simulink model "CAVE_MachE"  (R2024a)
settings: configuration reference "ConfigSetDesktopFixedStep" (kept outside this file)
PreLoadFcn:
  | VSS_BICYCLE=Simulink.Variant('Dual=0');
  | VSS_DUAL=Simulink.Variant('Dual=1');
  | Dual=1;
  | load('DriveCycle2.mat')
PostLoadFcn:
  | if any(exist('dsrtsu_mdlpostloadfcn', 'file') ~= 0), dsrtsu_mdlpostloadfcn('Execute', bdroot); end
InitFcn:
  | , if any(exist('rtifpga_mdlclblib', 'file') ~= 0), rtifpga_mdlclblib('Init', bdroot); end,
  | , if any(exist('dsmpb_private', 'file') ~= 0), dsmpb_private('dsmpb_mdlclblib', 'Init', bdroot); end,
  | load('DriveCycle2.mat')
model workspace (MAT data in the model file):
  Gas = 0.383333333333
undefined symbols (not defined in the file or in its folder): AccelCmd, ActTqLF_Nm_, ActTqLR_Nm_, ActTqRF_Nm_, ActTqRR_Nm_, BattChargeLimitMaxPwr, BattChargeLimitSocBpts, BattChargeLimitTbl, BattChrgCapcty, BattDischargeLimitSocBpts, BattDischargeLimitTbl, BattDischargeMaxPwr, BattNumCellsParallel, BattNumCellsSeries, BattOpenVoltCapBpts, BattOpenVoltTbl, BattResistSocBpts, BattResistTbl, BattResistTempBpts, BrakeMaxPrs, BrakeMaxTrq, ChassisDistCg2FrontAxle, ChassisDistCg2RearAxle, ChassisVehMass, CltchCmd, CoastDown, DecelCmd, DiffRatio, DiscIntNeverNeededParam, EnvGravCnst, EnvPrs, EnvTemp, FuelSpecificGrav, GearCmd, h, InitStates, lgSw, limitedMCT, MCT, MtrEffSpdBpts, MtrEffTbl, MtrEffTrqBpts, MtrPwrMax, MtrTrqMax, pMCT, Ref_speed, Ref_time, SteeringCmd, SupvsryCtrlRegenBrkCutOffTbl, SupvsryCtrlRegenSpdBpts, TestScnrioCycleNum, US06, VEH
libraries: VSIGenLib x65, simulink x54, etargetslib x38, dsmpblib x24, vehdynlibtire x12, autolibshared x9, vehdynlibsuspension x7, vehdynlibtirecommon x7, autolibutils x5, CarMaker4SL x4, VsrLibWheel x4, autolibpowerinfoutils x3
(part 3 of 14)

== system CAVE_MachE/Vehicle Under Test/Vehicle/Actuation and Outputs/Vehicle Accel Pedal Voltage Output ==
  APP_pct : Inport
  APP1Tbl : Lookup_n-D  NumberOfTableDimensions=1  BreakpointsForDimension1=[0 100]  Table=[16 78.8]  InternalRulePriority=Speed  RndMeth=Simplest
  APP2Tbl : Lookup_n-D  NumberOfTableDimensions=1  BreakpointsForDimension1=[0 100]  Table=[8 39.4]  InternalRulePriority=Speed  RndMeth=Simplest
  AccelPosition Bypass Enable : Constant  Value=0
  AccelPosition Manual Bypass [%] : Constant  Value=0
  Gain : Gain
  Gain1 : Gain
  Gain2 : Gain
  Gain3 : Gain  Gain=1/100
  Gain4 : Gain  Gain=1/100
  Product2 : Product
  Product3 : Product
  Rate Limiter : RateLimiter  RisingSlewLimit=50  FallingSlewLimit=-50  SampleTimeMode=inherited
  Switch2 : Switch  Criteria=u2 > Threshold  SaturateOnIntegerOverflow=off  InputSameDT=off
  Terminator2 : Terminator
  VRef : Constant  Value=5.01
  Voltage Out (1) : dsmpblib/Data Outport  Priority=-10000
      settings: SourceProductName=dSPACE Model Interface Package for Simulink (MIPS)
  Voltage Out (2) : dsmpblib/Data Outport  Priority=-10000
      settings: SourceProductName=dSPACE Model Interface Package for Simulink (MIPS)
  wires:
  Switch2/1 -> APP1Tbl/1, APP2Tbl/1, Gain2/1  "APP_CmdFinal_pct"
  APP_pct/1 -> Switch2/3
  AccelPosition Manual Bypass [%]/1 -> Rate Limiter/1
  AccelPosition Bypass Enable/1 -> Switch2/2
  Gain/1 -> Voltage Out (2)/1  "APP2_CmdFinal_V"
  Gain1/1 -> Voltage Out (1)/1  "APP1_CmdFinal_V"
  Gain2/1 -> Terminator2/1  "AccelPedal_CmdFinal_pct"
  Rate Limiter/1 -> Switch2/1
  VRef/1 -> Product2/2, Product3/1
  Gain4/1 -> Product3/2
  Product2/1 -> Gain1/1
  APP2Tbl/1 -> Gain4/1
  Gain3/1 -> Product2/1
  Product3/1 -> Gain/1
  APP1Tbl/1 -> Gain3/1

== system CAVE_MachE/Vehicle Under Test/Vehicle/Battery/Battery ==
  note: Thermal model is needed to estimated battery temperature. Ambient temperture is assumed.
  Bus Creator1 : BusCreator  Inputs=1
  Bus Selector : BusSelector  OutputSignals=BattSoc
  Bus Selector2 : BusSelector  OutputSignals=Curr
  Constant : Constant  Value=EnvTemp
  Lithium Ion Battery Pack1 : Subsystem  AncestorBlock=autolibdatasheetbattery/Datasheet Battery  mask(Datasheet Battery){CapacityCtrl=Parameter, OutputVlt=Unfiltered, BattChargeMax=BattChrgCapcty, Em=BattOpenVoltTbl, CapLUTBp=BattOpenVoltCapBpts, RInt=BattResistTbl, BattTempBp=BattResistTempBpts, CapSOCBp=BattResistSocBpts, Ns=BattNumCellsSeries, Np=BattNumCellsParallel, BattCapInit=InitStates(TestScnrioCycleNum).BattSoc*BattChrgCapcty, Tc=1/1000, Vinit=3.75*72, RefBlkName='autolibdatasheetbattery/Datasheet Battery'}
      mask prompts: CapacityCtrl "autoblks:autoblkDatasheetBattery:blkPrm_CapacityCtrl"; OutputVlt "autoblks:autoblkDatasheetBattery:blkPrm_OutputVlt"; BattChargeMax "autoblks:autoblkDatasheetBattery:blkPrm_BattChargeMax"; Em "autoblks:autoblkDatasheetBattery:blkPrm_Em"; CapLUTBp "autoblks:autoblkDatasheetBattery:blkPrm_CapLUTBp"; RInt "autoblks:autoblkDatasheetBattery:blkPrm_RInt"; BattTempBp "autoblks:autoblkDatasheetBattery:blkPrm_BattTempBp"; CapSOCBp "autoblks:autoblkDatasheetBattery:blkPrm_CapSOCBp"; Ns "autoblks:autoblkDatasheetBattery:blkPrm_Ns"; Np "autoblks:autoblkDatasheetBattery:blkPrm_Np"; BattCapInit "autoblks:autoblkDatasheetBattery:blkPrm_BattCapInit"; Tc "autoblks:autoblkDatasheetBattery:blkPrm_Tc"; Vinit "autoblks:autoblkDatasheetBattery:blkPrm_Vinit"
      mask help: autoblks:autoblkDatasheetBattery:blkDesc
      mask init:
      | autoicon('autolibdatasheetbattery',gcb,'Initialization');
      mask Help: eval('autoblkshelp(''pbbatterydatasheet'')');
      mask TypeOptions CapacityCtrl: autoblks:autoblkDatasheetBattery:blkCmb_CapacityCtrlExternalInput | autoblks:autoblkDatasheetBattery:blkCmb_CapacityCtrlParameter
      mask TypeOptions OutputVlt: autoblks:autoblkDatasheetBattery:blkCmb_OutputVltFiltered | autoblks:autoblkDatasheetBattery:blkCmb_OutputVltUnfiltered
      mask DialogControl Container3 Prompt: autoblks:autoblkDatasheetBattery:blkDlg_Container3
      mask DialogControl CapacityCtrl Prompt: Initial battery capacity:
      mask DialogControl OutputVlt Prompt: Output battery voltage:
      mask DialogControl ParameterGroupVar Prompt: autoblks:autoblkDatasheetBattery:blkDlg_ParameterGroupVar
      mask DialogControl BattChargeMax Prompt: Rated capacity at nominal temperature, BattChargeMax [Ah]:
      mask DialogControl Em Prompt: Open circuit voltage table data, Em [V]:
      mask DialogControl CapLUTBp Prompt: Open circuit voltage breakpoints 1, CapLUTBp []:
      mask DialogControl RInt Prompt: Internal resistance table data, RInt [Ohms]:
      mask DialogControl BattTempBp Prompt: Battery temperature breakpoints 1, BattTempBp [K]:
      mask DialogControl CapSOCBp Prompt: Battery capacity breakpoints 2, CapSOCBp []:
      mask DialogControl Ns Prompt: Number of cells in series, Ns []:
      mask DialogControl Np Prompt: Number of cells in parallel, Np []:
      mask DialogControl BattCapInit Prompt: Initial battery capacity, BattCapInit [Ah]:
      mask DialogControl Tc Prompt: Output battery voltage time constant, Tc [s]:
      mask DialogControl Vinit Prompt: Output battery voltage initial value, Vinit [V]:
      mask Display:
      | IconInfo = autoicon('autolibdatasheetbattery', gcb, 'DrawCommands');
      | 
      | image(IconInfo.image, IconInfo.position);
      | 
      | for i = 1:numel(IconInfo.lconn)
      |     port_label('lconn', i, IconInfo.lconn{i})
      | end
      | 
      | for j = 1:numel(IconInfo.rconn)
      |     port_label('rconn', j, IconInfo.rconn{j})
      | end
      | 
      | for k = 1:numel(IconInfo.input)
      |     port_label('input', k, IconInfo.input{k})
      | end
      | 
      | for m = 1:numel(IconInfo.output)
      |     port_label('output', m, IconInfo.output{m})
      | end
  Two-Way Connection1 : TwoWayConnection
  Batt : PMIOPort  Side=Right
  BattSoc : Outport
  BattCurr : Outport  Port=2  Unit=A
  BattVolt : Outport  Port=3  Unit=V
  wires:
  Bus Selector2/1 -> Lithium Ion Battery Pack1/1(BattCurr), BattCurr/1  "<Curr>"
  Lithium Ion Battery Pack1/2(BattVolt) -> BattVolt/1, Bus Creator1/1  "Volt"
  Bus Creator1/1 -> Two-Way Connection1/1
  Constant/1 -> Lithium Ion Battery Pack1/2(BattTemp)
  Bus Selector/1 -> BattSoc/1  "<BattSoc>"
  Lithium Ion Battery Pack1/1(Info) -> Bus Selector/1
  Two-Way Connection1/1 -> Bus Selector2/1
  connections:
  Batt/RConn1 -- Two-Way Connection1/RConn1

== system CAVE_MachE/Vehicle Under Test/Vehicle/Battery/Subsystem1 ==
  BattSoc : Inport
  BattCurr : Inport  Port=2
  BattVolt : Inport  Port=3
  Bus Creator : BusCreator  Inputs=3
  Batt : Outport
  wires:
  BattSoc/1 -> Bus Creator/1  "BattSoc"
  BattCurr/1 -> Bus Creator/2  "BattCurr"
  Bus Creator/1 -> Batt/1  "Batt"
  BattVolt/1 -> Bus Creator/3  "BattVolt"

== system CAVE_MachE/Vehicle Under Test/Vehicle/Driver and Drive Cycle/Driver and PI with FF Control ==
  Vehicle_Spd_kph : Inport
  Vehicle_SpdDmd_kph : Inport  Port=2
  Bus Creator : BusCreator  Inputs=6
  Constant : Constant
  Memory1 : Memory
  Memory2 : Memory
  SpdSat : Saturate  UpperLimit=190  LowerLimit=-5
  Speed controller set : Subsystem
  km to miles : Gain  Gain=1/1.609344
  DriverBus : Outport
  wires:
  Vehicle_SpdDmd_kph/1 -> Memory1/1
  Constant/1 -> Bus Creator/1  "Drive"
  SpdSat/1 -> Speed controller set/1(RefSpd [km/hr]), km to miles/1, Bus Creator/5  "RefSpd [km/hr]"
  Bus Creator/1 -> DriverBus/1  "DriverBus"
  Vehicle_Spd_kph/1 -> Memory2/1
  km to miles/1 -> Bus Creator/6  "RefSpd [mph]"
  Memory1/1 -> SpdSat/1
  Memory2/1 -> Speed controller set/2(VehSpd)
  Speed controller set/1(Out1) -> Bus Creator/2
  Speed controller set/2(Out2) -> Bus Creator/3
  Speed controller set/3(Out3) -> Bus Creator/4

== system CAVE_MachE/Vehicle Under Test/Vehicle/Driver and Drive Cycle/Get Cycle Clock Time ==
  Cycle Trigger : Inport
  Add1 : Sum  Inputs=+-
  Clock1 : Clock
  Clock2 : Clock
  Data Type Conversion : DataTypeConversion  OutDataTypeStr=double  SaturateOnIntegerOverflow=off  RndMeth=Floor
  Memory4 : Memory
  Switch : Switch  Criteria=u2 > Threshold  SaturateOnIntegerOverflow=off  InputSameDT=off
  tCycle : Outport
  wires:
  Switch/1 -> Add1/2, Memory4/1
  Clock1/1 -> Add1/1
  Clock2/1 -> Switch/3
  Add1/1 -> tCycle/1  "tCycle"
  Memory4/1 -> Switch/1
  Cycle Trigger/1 -> Data Type Conversion/1
  Data Type Conversion/1 -> Switch/2

== system CAVE_MachE/Vehicle Under Test/Vehicle/Front Wheel Drive/Ideal Diff ==
  DrvShfTrq : Inport
  Omega : Inport  Port=2
  Add : Sum
  Add1 : Sum
  Bus Creator1 : BusCreator  Inputs=2
  Bus Creator2 : BusCreator  Inputs=2
  Bus Creator3 : BusCreator  Inputs=2
  Bus Creator4 : BusCreator  Inputs=4
  Bus to Vector : BusToVector
  Constant : Constant  Value=0
  Demux : Demux  Outputs=[2,2]
  Demux1 : Demux  Outputs=2
  Gain1 : Gain  Gain=0.5
  Gain2 : Gain  Gain=DiffRatio
  Gain3 : Gain  Gain=DiffRatio
  Gain4 : Gain  Gain=0.5
  Memory : Memory
  Memory1 : Memory
  Power Bus : Subsystem
  Terminator : Terminator
  Terminator1 : Terminator
  Vector Concatenate : Concatenate  NumInputs=4
  Diff : Outport  VectorParamsAs1DForOutWhenUnconnected=off
  AxlTrq : Outport  Port=2  VectorParamsAs1DForOutWhenUnconnected=off
  PropShaftSpd : Outport  Port=3  VectorParamsAs1DForOutWhenUnconnected=off
  wires:
  Demux1/2 -> [Axl2Spd], Add1/2
  Vector Concatenate/1 -> AxlTrq/1
  Gain4/1 -> [Axl1Trq], Add/1, Vector Concatenate/1, [Axl2Trq], Add/2, Vector Concatenate/2  "T_FL"
  DrvShfTrq/1 -> [DriveshftTrq], Bus to Vector/1
  [DriveshftTrq] -> Power Bus/1(DriveshftTrq), Bus Creator1/1  "DriveshftTrq"
  [Axl1Spd] -> Bus Creator2/2  "Axl1Spd"
  Demux/1 -> Demux1/1
  Add1/1 -> Gain1/1
  Bus Creator4/1 -> Diff/1
  Add/1 -> Terminator/1  "AxlTrqLump"
  [Axl2Trq] -> Bus Creator3/1  "Axl2Trq"
  Omega/1 -> Demux/1
  Memory/1 -> Gain3/1
  Bus to Vector/1 -> Memory/1
  Bus Creator3/1 -> Bus Creator4/3  "Axl2"
  Bus Creator2/1 -> Bus Creator4/2  "Axl1"
  Bus Creator1/1 -> Bus Creator4/1  "Driveshft"
  [DriveshftSpd] -> Bus Creator1/2, Power Bus/2(Speed)  "Speed"
  Gain2/1 -> Memory1/1  "Spd"
  Constant/1 -> Vector Concatenate/4, Vector Concatenate/3  "T_RR"
  Demux1/1 -> [Axl1Spd], Add1/1
  Memory1/1 -> PropShaftSpd/1, [DriveshftSpd]
  Gain3/1 -> Gain4/1
  [Axl1Trq] -> Bus Creator2/1  "Axl1Trq"
  Power Bus/1(PwrInfo) -> Bus Creator4/4
  Gain1/1 -> Gain2/1
  [Axl2Spd] -> Bus Creator3/2  "Axl2Spd"
  Demux/2 -> Terminator1/1

== system CAVE_MachE/Vehicle Under Test/Vehicle/Front Wheel Drive/Ideal Diff AWD ==
  DrvShfTrq : Inport
  Omega : Inport  Port=2
  Add : Sum
  Add1 : Sum  Inputs=++++
  Bus Creator1 : BusCreator  Inputs=2
  Bus Creator2 : BusCreator  Inputs=2
  Bus Creator3 : BusCreator  Inputs=2
  Bus Creator4 : BusCreator  Inputs=4
  Bus to Vector : BusToVector
  Demux : Demux  Outputs=[2,2]
  Demux1 : Demux  Outputs=2
  Demux2 : Demux  Outputs=2
  Gain1 : Gain  Gain=0.25
  Gain2 : Gain  Gain=DiffRatio
  Gain3 : Gain  Gain=DiffRatio
  Gain4 : Gain  Gain=0.25
  Memory : Memory
  Memory1 : Memory
  Power Bus : Subsystem
  Terminator : Terminator
  Vector Concatenate : Concatenate  NumInputs=4
  Diff : Outport  VectorParamsAs1DForOutWhenUnconnected=off
  AxlTrq : Outport  Port=2  VectorParamsAs1DForOutWhenUnconnected=off
  PropShaftSpd : Outport  Port=3  VectorParamsAs1DForOutWhenUnconnected=off
  wires:
  Power Bus/1(PwrInfo) -> Bus Creator4/4
  Demux1/2 -> [Axl2Spd], Add1/2
  Gain4/1 -> [Axl4Trq], Vector Concatenate/4, [Axl3Trq], Vector Concatenate/3, [Axl1Trq], Add/1, Vector Concatenate/1, [Axl2Trq], Add/2, Vector Concatenate/2  "T_RR"
  Demux/2 -> Demux2/1
  Vector Concatenate/1 -> AxlTrq/1
  Gain1/1 -> Gain2/1
  Gain3/1 -> Gain4/1
  [Axl1Trq] -> Bus Creator2/1  "Axl1Trq"
  Bus to Vector/1 -> Memory/1
  Gain2/1 -> Memory1/1  "Spd"
  Memory/1 -> Gain3/1
  Bus Creator2/1 -> Bus Creator4/2  "Axl1"
  Memory1/1 -> PropShaftSpd/1, [DriveshftSpd]
  Demux1/1 -> [Axl1Spd], Add1/1
  [DriveshftSpd] -> Bus Creator1/2, Power Bus/2(Speed)  "Speed"
  Bus Creator4/1 -> Diff/1
  [Axl2Spd] -> Bus Creator3/2  "Axl2Spd"
  Bus Creator1/1 -> Bus Creator4/1  "Driveshft"
  Add/1 -> Terminator/1  "AxlTrqLump"
  [Axl1Spd] -> Bus Creator2/2  "Axl1Spd"
  [Axl2Trq] -> Bus Creator3/1  "Axl2Trq"
  DrvShfTrq/1 -> [DriveshftTrq], Bus to Vector/1
  Demux/1 -> Demux1/1
  Bus Creator3/1 -> Bus Creator4/3  "Axl2"
  [DriveshftTrq] -> Power Bus/1(DriveshftTrq), Bus Creator1/1  "DriveshftTrq"
  Add1/1 -> Gain1/1
  Omega/1 -> Demux/1
  Demux2/1 -> Add1/3
  Demux2/2 -> Add1/4

== system CAVE_MachE/Vehicle Under Test/Vehicle/Front Wheel Drive/Real Diff ==
  DrvShfTrq : Inport
  Omega : Inport  Port=2
  Bus Creator1 : BusCreator  Inputs=2
  Bus Creator2 : BusCreator  Inputs=2
  Bus Creator3 : BusCreator  Inputs=2
  Bus Creator4 : BusCreator  Inputs=4
  Constant : Constant  Value=0
  Demux : Demux  Outputs=[2,2]
  Demux1 : Demux  Outputs=2
  DiffPress : Constant  Value=0
  Limited Slip Differential : autolibshareddiff/Limited Slip Differential  DiffEffModelPopup=Constant  InterpMethod=Linear point-slope  extTamb=off  shaftSwitchMask=To the left of center-line  Ndiff=7.05  Jd=0.025  bd=1e-3  Jw1=0.01  bw1=1e-3  Jw2=0.01  bw2=1e-3  omegaw1o=0  omegaw2o=0  eta=0.98  eta_tbl=reshape([0.64 0.76 0.8 0.81 0.83 0.84 0.84 0.56 0.73 0.78 0.8 0.83 0.84 0.84 0.54 0.71 0.77 0.8 0.82 0.84 0.84 0.53 0.71 0.77 0.8 0.83 0.84 0.84 0.51 0.71 0.77 0.8 0.83 0.84 0.85 0.52 0.7 0.77 0.8 0.83 0.84 0.85 0.51 0.71 0.76 0.79 0.83 0.84 0.85 0.5 0.69 0.76 0.79 0.82 0.84 0.85 0.45 0.68 0.75 0.78 0.82 0.84 0.85 0.43 0.67 0.74 0.78 0.81 0.83 0.84 0.38 0.63 0.71 0.75 0.8 0.82 0.83 0.81 0.86 0.88 0.89 0.89 0.89 0.9 0.77 0.85 0.87 0.88 0.89 0.9 0.9 0.72 0.82 0.86 0.87 0.88 0.89 0.9 0.68 0.8 0.84 0.86 0.88 0.89 0.89 0.67 0.8 0.84 0.86 0.88 0.89 0.9 0.67 0.8 0.84 0.86 0.88 0.89 0.9 0.65 0.8 0.84 0.86 0.88 0.89 0.9 0.64 0.79 0.83 0.86 0.88 0.89 0.9 0.63 0.78 0.83 0.86 0.88 0.89 0.9 0.59 0.76 0.82 0.85 0.87 0.89 0.9 0.53 0.73 0.8 0.83 0.86 0.88 0.89], 7, 11, 2)  Trq_bpts=[25, 50, 75, 100, 150, 200, 250]  omega_bpts=[52.4 78.5 105 131 157 183 209 262 314 419 524]  Temp_bpts=[290 358]  Tamb=297.15  couplingType=Pre-loaded ideal clutch  Ndisks=8  Reff=.08  Fc=1000  muc=[.16 0.13 0.115 0.11 0.105 0.1025 0.10125 .10125]  dw=[0 10 20 40 60 80 100 1000]  Tdw=[-100, -90, -50, -5, 0, 5, 50, 90, 100]  dwT=[-200, -175, -100, - 50, 0, 50, 100, 175, 200]  TTin=[-200 -175 -100 - 50 0 50 100 175 200]  Tin=[-200 -175 -100 - 50 0 50 100 175 200]  tauC=.04  IdealInterpMethod=Linear point-slope  IdealExtrapMethod=Linear  TdwInterpMethod=Flat  TdwExtrapMethod=Clip  TTinInterpMethod=Flat  TTinExtrapMethod=Clip  maxAbsSpd=5e3  aMode=2
      settings: LibrarySourceBlock=vdynlib/Powertrain/Drivetrain/Final Drive Unit/Limited Slip Differential
  Power Bus : Subsystem
  Terminator : Terminator
  Terminator1 : Terminator
  Terminator3 : Terminator
  Torsional Compliance1 : autolibsharedcoupling/Torsional Compliance  port_config=Simulink  extInfo=off  k=10000  b=400  theta_o=0  domega_o=0  omega_c=300  blkID=0  aMode=2
      settings: LibrarySourceBlock=vdynlib/Powertrain/Drivetrain/Couplings/Torsional Compliance
  Torsional Compliance2 : autolibsharedcoupling/Torsional Compliance  port_config=Simulink  extInfo=off  k=10000  b=400  theta_o=0  domega_o=0  omega_c=300  blkID=0  aMode=2
      settings: LibrarySourceBlock=vdynlib/Powertrain/Drivetrain/Couplings/Torsional Compliance
  Vector Concatenate : Concatenate  NumInputs=4
  Vector Concatenate1 : Concatenate  NumInputs=4
  Diff : Outport  VectorParamsAs1DForOutWhenUnconnected=off
  AxlTrq : Outport  Port=2  VectorParamsAs1DForOutWhenUnconnected=off
  PropShaftSpd : Outport  Port=3  VectorParamsAs1DForOutWhenUnconnected=off
  wires:
  Limited Slip Differential/3 -> [Axl1Spd], Torsional Compliance2/1
  Demux1/1 -> Torsional Compliance2/2
  Limited Slip Differential/1 -> Terminator/1
  DrvShfTrq/1 -> [DriveshftTrq], Limited Slip Differential/1
  Limited Slip Differential/4 -> [Axl2Spd], Torsional Compliance1/1
  Demux1/2 -> Torsional Compliance1/2
  Demux/1 -> Demux1/1
  Torsional Compliance1/1 -> Limited Slip Differential/3
  Torsional Compliance2/1 -> Limited Slip Differential/2
  Demux/2 -> Terminator1/1
  Constant/1 -> Vector Concatenate/4, Vector Concatenate/3  "T_RR"
  Torsional Compliance1/2 -> [Axl2Trq], Vector Concatenate/2  "T_FR"
  Torsional Compliance2/2 -> [Axl1Trq], Vector Concatenate/1  "T_FL"
  Omega/1 -> Demux/1
  Vector Concatenate/1 -> AxlTrq/1
  Vector Concatenate1/1 -> Terminator3/1
  DiffPress/1 -> Vector Concatenate1/4, Vector Concatenate1/3, Vector Concatenate1/1, Vector Concatenate1/2
  [DriveshftTrq] -> Power Bus/1(DriveshftTrq), Bus Creator1/1  "DriveshftTrq"
  [Axl1Spd] -> Bus Creator2/2  "Axl1Spd"
  [Axl2Trq] -> Bus Creator3/1  "Axl2Trq"
  Bus Creator4/1 -> Diff/1
  [Axl2Spd] -> Bus Creator3/2  "Axl2Spd"
  [DriveshftSpd] -> Bus Creator1/2, Power Bus/2(Speed)  "Speed"
  Bus Creator1/1 -> Bus Creator4/1  "Driveshft"
  [Axl1Trq] -> Bus Creator2/1  "Axl1Trq"
  Power Bus/1(PwrInfo) -> Bus Creator4/4
  Bus Creator2/1 -> Bus Creator4/2  "Axl1"
  Bus Creator3/1 -> Bus Creator4/3  "Axl2"
  Limited Slip Differential/2 -> [DriveshftSpd], PropShaftSpd/1

== system CAVE_MachE/Vehicle Under Test/Vehicle/Powertrain Supervisory Controller /Engine Torque Command ==
  AccelCmdIn : Inport
  DecelCmdIn : Inport  Port=2
  DriverGearCmdIn : Inport  Port=3
  VehSpd : Inport  Port=4
  BattSoc : Inport  Port=5
  MtrSpd : Inport  Port=6
  Accel Pedal to Traction Wheel Torque Request1 : Subsystem
  Battery Management System : Subsystem
  Motor Torque Arbitration and Power Management : Subsystem
  Series Regen Braking : Subsystem  InitFcn=%[~]=autosharedicon('autolibutils',gcb,0);  VariantControl=Variant
  MtrTrqCmd : Outport
  AccelCmd : Outport  Port=2
  BrkCmd : Outport  Port=3
  DriverGearCmd : Outport  Port=4
  wires:
  DecelCmdIn/1 -> Series Regen Braking/4("DecelCmd ")  "DecelPdl"
  DriverGearCmdIn/1 -> DriverGearCmd/1
  [AccelPdl] -> Motor Torque Arbitration and Power Management/2(AccelPdl)
  MtrSpd/1 -> [MotSpd], Series Regen Braking/3(MotSpd)  "MotSpd"
  AccelCmdIn/1 -> AccelCmd/1, Accel Pedal to Traction Wheel Torque Request1/1(AccelPdl), [AccelPdl]
  VehSpd/1 -> [VehSpd], Series Regen Braking/2(VehSpd)  "VehSpd"
  BattSoc/1 -> Battery Management System/1(SOC), Series Regen Braking/1(BattSoc)  "SOC"
  Battery Management System/1(BattPwrDischrgLmt) -> Motor Torque Arbitration and Power Management/3(BattPwrDisChrgLmt)  "BattPwrDischrgLmt"
  Series Regen Braking/2(" BrkCmd") -> BrkCmd/1  "BrkCmd"
  Battery Management System/2(BattPwrChrgLmt) -> Motor Torque Arbitration and Power Management/4("BattPwrChrgLmt ")  "BattPwrChrgLmt"
  Series Regen Braking/1(" MotTrqCmdRegen") -> Motor Torque Arbitration and Power Management/6(MotTrqCmdRegen)  "MotTrqCmdRegen"
  [MotSpd] -> Motor Torque Arbitration and Power Management/5(MotSpd)
  Motor Torque Arbitration and Power Management/1(MotTrqCmdFinal) -> MtrTrqCmd/1  "MotTrqCmd"
  [VehSpd] -> Accel Pedal to Traction Wheel Torque Request1/2(MotSpd)
  Accel Pedal to Traction Wheel Torque Request1/1(TrqCmd) -> Motor Torque Arbitration and Power Management/1(MotTrqCmdTrac)

== system CAVE_MachE/Vehicle Under Test/Vehicle/Powertrain Supervisory Controller /Subsystem1 ==
  MtrTrqCmd : Inport
  AccelCmd : Inport  Port=2
  BrkCmd : Inport  Port=3
  DriverGearCmd : Inport  Port=4
  SteeringCmd : Inport  Port=5
  Bus Creator : BusCreator  Inputs=5
  SupvsryCtrl : Outport
  wires:
  MtrTrqCmd/1 -> Bus Creator/1  "MtrTrqCmd"
  Bus Creator/1 -> SupvsryCtrl/1  "SupvsryCtrl"
  AccelCmd/1 -> Bus Creator/2  "AccelCmd"
  BrkCmd/1 -> Bus Creator/3  "BrkCmd"
  DriverGearCmd/1 -> Bus Creator/4  "DriverGearCmd"
  SteeringCmd/1 -> Bus Creator/5  "SteeringCmd"

== system CAVE_MachE/Vehicle Under Test/Vehicle/Powertrain Supervisory Controller /Subsystem4 ==
  Driver : Inport
  Chassis : Inport  Port=2
  Batt : Inport  Port=3
  Mtr : Inport  Port=4
  Bus Selector : BusSelector  OutputSignals=AccelCmd,DecelCmd,GearCmd
  Bus Selector1 : BusSelector  OutputSignals=VehSpd
  Bus Selector2 : BusSelector  OutputSignals=BattSoc
  Bus Selector3 : BusSelector  OutputSignals=MtrSpd
  AccelCmd : Outport  VectorParamsAs1DForOutWhenUnconnected=off
  DecelCmd : Outport  Port=2  VectorParamsAs1DForOutWhenUnconnected=off
  DriverGearCmd : Outport  Port=3  VectorParamsAs1DForOutWhenUnconnected=off
  VehSpd : Outport  Port=4  VectorParamsAs1DForOutWhenUnconnected=off
  BattSoc : Outport  Port=5  VectorParamsAs1DForOutWhenUnconnected=off
  MtrSpd : Outport  Port=6  VectorParamsAs1DForOutWhenUnconnected=off
  wires:
  Driver/1 -> Bus Selector/1
  Bus Selector/1 -> AccelCmd/1  "<AccelCmd>"
  Bus Selector/3 -> DriverGearCmd/1  "<GearCmd>"
  Chassis/1 -> Bus Selector1/1
  Bus Selector1/1 -> VehSpd/1  "<VehSpd>"
  Bus Selector/2 -> DecelCmd/1  "<DecelCmd>"
  Batt/1 -> Bus Selector2/1
  Bus Selector2/1 -> BattSoc/1  "<BattSoc>"
  Mtr/1 -> Bus Selector3/1
  Bus Selector3/1 -> MtrSpd/1  "<MtrSpd>"

== system CAVE_MachE/Vehicle Under Test/Vehicle/Rototest and ORNL Interface/DummyPT ==
  WhlSpeedIn : Inport
  APPToTorque : Lookup_n-D  NumberOfTableDimensions=1  BreakpointsForDimension1=[0 100]  Table=[0 184]  InternalRulePriority=Speed  RndMeth=Simplest
  APPToTorque1 : Lookup_n-D  NumberOfTableDimensions=1  BreakpointsForDimension1=[0 100]  Table=[0 184]  InternalRulePriority=Speed  RndMeth=Simplest
  APP_pct : Constant  Value=0
  BPP_pct : Constant  Value=0
  FDR : Gain  Gain=3.18
  Flip : Gain  Gain=-1
  Gear : Product
  Memory : Memory
  NissanTrans : Lookup_n-D  NumberOfTableDimensions=1  BreakpointsForDimension1=[0 5 10 15 25 34 45 55]  Table=[5.25 3.03 1.95 1.46 1.22 1.00 0.81 0.67]  ExtrapMethod=Clip  InternalRulePriority=Speed  RndMeth=Simplest
  Sum : Sum  Inputs=++|
  WheelRadius : Gain  Gain=0.3235
  kph2mph : Gain  Gain=0.621
  mps2kph : Gain  Gain=3.6
  WheelTorqueOut : Outport
  wires:
  kph2mph/1 -> NissanTrans/1  "Speed_mph"
  APPToTorque/1 -> Sum/1  "APPTorque"
  mps2kph/1 -> kph2mph/1  "Speed_kph"
  BPP_pct/1 -> APPToTorque1/1
  NissanTrans/1 -> Gear/2  "Gear"
  Gear/1 -> FDR/1  "TransTorqueOut"
  APPToTorque1/1 -> Flip/1
  Flip/1 -> Sum/2  "BPPTorque"
  APP_pct/1 -> APPToTorque/1
  Sum/1 -> Gear/1  "TorqueTotal"
  WheelRadius/1 -> mps2kph/1  "Speed_mps"
  FDR/1 -> Memory/1  "WheelTorqueOut"
  WhlSpeedIn/1 -> WheelRadius/1
  Memory/1 -> WheelTorqueOut/1

== system CAVE_MachE/Vehicle Under Test/Vehicle/Rototest and ORNL Interface/Format CM Powertrain Signals ==
  note: Can Bypass with my own brake model
  BrakingTorques : Inport
  RotoWheelSpd : Inport  Port=2
  AxlTrq : Inport  Port=3
  MaxRegen : Inport  Port=4
  Bus Creator1 : BusCreator  Inputs=42
  Bus Selector2 : BusSelector  OutputSignals=Brake IF Trq_WB FL,Brake IF Trq_WB FR,Brake IF Trq_WB RL,Brake IF Trq_WB RR
  BusCreator2 : BusCreator  Inputs=42
  Demux : Demux
  Demux1 : Demux  Outputs=42
      settings: DisplayOption=none
  Demux2 : Demux
  Discrete-Time Integrator{4..7} (4 alike) : DiscreteIntegrator  IntegratorMethod=Integration: Backward Euler  SampleTime=0.001  ICPrevOutput=DiscIntNeverNeededParam  ICPrevScaledInput=DiscIntNeverNeededParam
  Gain{5..8} (4 alike) : Gain  Gain=-1
  Ground{2..5} (4 alike) : Ground
  Ignition : Constant
  Memory{1..4} (4 alike) : Memory
  Operation Error : Constant  Value=4
  Operation State Driving : Constant  Value=4
  Product{1..4} (4 alike) : Product  RndMeth=Zero
  Saturation{1..4} (4 alike) : Saturate  UpperLimit=1  LowerLimit=-1
  Zero{1..5} (5 alike) : Constant  Value=0
  PowerTrainOutIdeal : Outport
  wires:
  Saturation4/1 -> Product4/2
  Demux1/3 -> BusCreator2/3  "PT IF OperationError"
  Demux1/2 -> BusCreator2/2  "PT IF OperationState"
  Demux1/40 -> BusCreator2/40  "PT IF WRR Trq_Supp2WC"
  Demux1/9 -> BusCreator2/9  "PT IF Trq_Supp2Bdy1B x"
  Discrete-Time Integrator6/1 -> Bus Creator1/29  "PT WRL rot"
  Demux1/1 -> BusCreator2/1  "PT IF Ignition"
  MaxRegen/1 -> Bus Creator1/28, Bus Creator1/21
  BusCreator2/1 -> PowerTrainOutIdeal/1
  Operation State Driving/1 -> Bus Creator1/2
  Gain8/1 -> Bus Creator1/38
  Demux1/16 -> BusCreator2/16  "PT IF WFL rotv"
  Demux1/21 -> BusCreator2/21  "PT IF WFL Trq_BrakeReg_max"
  Ground2/1 -> Bus Creator1/7
  Demux1/23 -> BusCreator2/23  "PT IF WFR rotv"
  Demux1/14 -> BusCreator2/14  "PT IF DL_iDiff_mean"
  Demux1/4 -> BusCreator2/4  "PT IF GearNo"
  Demux1/17 -> BusCreator2/17  "PT IF WFL Trq_B2W"
  Product3/1 -> Gain5/1
  Demux1/5 -> BusCreator2/5  "PT IF Engine_rotv"
  Demux1/11 -> BusCreator2/11  "PT IF Trq_Supp2Bdy1B z"
  Demux1/12 -> BusCreator2/12  "PT IF Trq_Supp2BdyEng x"
  Demux1/7 -> BusCreator2/7  "PT IF Trq_Supp2Bdy1 y"
  Discrete-Time Integrator5/1 -> Bus Creator1/22  "PT WFR rot"
  Demux1/42 -> BusCreator2/42  "PT IF WRR Trq_BrakeReg_max"
  Gain5/1 -> Bus Creator1/17
  Demux1/18 -> BusCreator2/18  "PT IF WFL Trq_Drive"
  Demux1/8 -> BusCreator2/8  "PT IF Trq_Supp2Bdy1 z"
  Demux1/38 -> BusCreator2/38  "PT IF WRR Trq_B2W"
  Memory4/1 -> Saturation4/1
  Demux1/10 -> BusCreator2/10  "PT IF Trq_Supp2Bdy1B y"
  Demux1/27 -> BusCreator2/27  "PT IF WFR Trq_BrakeReg"
  Demux1/24 -> BusCreator2/24  "PT IF WFR Trq_B2W"
  Demux1/25 -> BusCreator2/25  "PT IF WFR Trq_Drive"
  Demux1/26 -> BusCreator2/26  "PT IF WFR Trq_Supp2WC"
  Demux1/13 -> BusCreator2/13  "PT IF Trq_Supp2BdyEng y"
  Demux1/15 -> BusCreator2/15  "PT IF WFL rot"
  Bus Selector2/2 -> Product1/1  "<Brake IF Trq_WB FR>"
  Memory3/1 -> Saturation3/1
  Demux1/19 -> BusCreator2/19  "PT IF WFL Trq_Supp2WC"
  Demux1/22 -> BusCreator2/22  "PT IF WFR rot"
  Demux1/29 -> BusCreator2/29  "PT IF WRL rot"
  Demux1/33 -> BusCreator2/33  "PT IF WRL Trq_Supp2WC"
  Demux1/30 -> BusCreator2/30  "PT IF WRL rotv"
  Demux1/28 -> BusCreator2/28  "PT IF WFR Trq_BrakeReg_max"
  Demux1/35 -> BusCreator2/35  "PT IF WRL Trq_BrakeReg_max"
  Demux1/39 -> BusCreator2/39  "PT IF WRR Trq_Drive"
  Zero4/1 -> Bus Creator1/33, Bus Creator1/34, Bus Creator1/35
  Demux1/34 -> BusCreator2/34  "PT IF WRL Trq_BrakeReg"
  Demux1/37 -> BusCreator2/37  "PT IF WRR rotv"
  Demux1/31 -> BusCreator2/31  "PT IF WRL Trq_B2W"
  Demux1/32 -> BusCreator2/32  "PT IF WRL Trq_Drive"
  Demux1/36 -> BusCreator2/36  "PT IF WRR rot"
  Zero3/1 -> Bus Creator1/26, Bus Creator1/27
  Demux/4 -> Memory4/1, Discrete-Time Integrator7/1, Bus Creator1/37  "rotv RR"
  Zero2/1 -> Bus Creator1/19, Bus Creator1/20
  Zero1/1 -> Bus Creator1/5, Bus Creator1/4, Bus Creator1/12, Bus Creator1/14, Bus Creator1/13, Bus Creator1/11, Bus Creator1/10, Bus Creator1/9, Bus Creator1/8
  Demux1/20 -> BusCreator2/20  "PT IF WFL Trq_BrakeReg"
  Product2/1 -> Gain7/1
  Discrete-Time Integrator4/1 -> Bus Creator1/15  "PT WFL rot"
  Demux/2 -> Memory1/1, Discrete-Time Integrator5/1, Bus Creator1/23  "rotv FR"
  Discrete-Time Integrator7/1 -> Bus Creator1/36  "PtT WRR rot"
  Zero5/1 -> Bus Creator1/40, Bus Creator1/41, Bus Creator1/42
  Demux1/6 -> BusCreator2/6  "PT IF Trq_Supp2Bdy1 x"
  Demux1/41 -> BusCreator2/41  "PT IF WRR Trq_BrakeReg"
  BrakingTorques/1 -> Bus Selector2/1
  Operation Error/1 -> Bus Creator1/3
  Demux/3 -> Memory2/1, Discrete-Time Integrator6/1, Bus Creator1/30  "rotv RL"
  Memory1/1 -> Saturation1/1
  Ground4/1 -> Bus Creator1/6
  Bus Selector2/1 -> Product3/1  "<Brake IF Trq_WB FL>"
  Gain6/1 -> Bus Creator1/24
  Ignition/1 -> Bus Creator1/1  "PT Ignition"
  Memory2/1 -> Saturation2/1
  Saturation1/1 -> Product1/2
  Bus Selector2/3 -> Product2/1  "<Brake IF Trq_WB RL>"
  Gain7/1 -> Bus Creator1/31
  Demux/1 -> Memory3/1, Discrete-Time Integrator4/1, Bus Creator1/16  "rotv FL"
  Product4/1 -> Gain8/1
  Bus Creator1/1 -> Demux1/1
  Saturation2/1 -> Product2/2
  Product1/1 -> Gain6/1
  Bus Selector2/4 -> Product4/1  "<Brake IF Trq_WB RR>"
  Saturation3/1 -> Product3/2
  RotoWheelSpd/1 -> Demux/1
  AxlTrq/1 -> Demux2/1
  Demux2/1 -> Bus Creator1/18  "TrqDrv FL"
  Demux2/2 -> Bus Creator1/25  "TrqDrv FR"
  Demux2/3 -> Bus Creator1/32  "TrqDrv RL"
  Demux2/4 -> Bus Creator1/39  "TrqDrv RR"

== system CAVE_MachE/Vehicle Under Test/Vehicle/Rototest and ORNL Interface/From Rototest ==
  Input : Inport
  Bus Creator : BusCreator  Inputs=30
  Bus Selector1 : BusSelector  OutputSignals=ActSpLF_rpm,ActSpRF_rpm,ActSpLR_rpm,ActSpRR_rpm
  Mux1 : Mux
  RotoTestEthRX : Subsystem  AncestorBlock=VSIGenLib/RotoTestEthRX
      mask Display:
      | color('white')
      | disp('RotTestEthTx')
      | port_label('output', 1, 'ID')
      | port_label('output', 2, 'ProtocolVer')
      | port_label('output', 3, 'ActTqLF (Nm)')
      | port_label('output', 4, 'RefRR_NmORrpm')
      | port_label('output', 5, 'ActTempLF (C)')
      | port_label('output', 6, 'ActTqRF (Nm)')
      | port_label('output', 7, 'ActSpRF (rpm)')
      | port_label('output', 8, 'ActTempRF (C)')
      | port_label('output', 9, 'ActTqLR (Nm)')
      | port_label('output', 10, 'ActSpLR (rpm)')
      | port_label('output', 11, 'ActTempLR (C)')
      | port_label('output', 12, 'ActTqRR (Nm)')
      | port_label('output', 13, 'ActSpRR (rpm)')
      | port_label('output', 14, 'ActTempRR (Nm)')
      | port_label('output', 15, 'RefLF (Nm)')
      | port_label('output', 16, 'RefRF (rpm)')
      | port_label('output', 17, 'RefLR (Nm)')
      | port_label('output', 18, 'RefRR (Nm)')
      | port_label('output', 19, 'UnitsStatusLF (enum)')
      | port_label('output', 20, 'UnitsStatusRF (enum)')
      | port_label('output', 21, 'UnitsStatusLR (enum)')
      | port_label('output', 22, 'UnitsStatusRR (enum)')
      | port_label('output', 23, 'WatchdogCnt (int)')
      | port_label('output', 24, 'FaultActive (enum)')
      | port_label('output', 25, 'WarningsActive (enum)')
      | port_label('output', 26, 'SpTqRR (enum)')
      | port_label('output', 27, 'SpTqLR (enum)')
      | port_label('output', 28, 'SpTqRF (enum)')
      | port_label('output', 29, 'SpTqLF (enum)')
      | port_label('output', 30, 'SystemActive (bool)')
  SpdAct : Outport
  AxlTrq : Outport  Port=2
  wires:
  RotoTestEthRX/8(ActTempRF_C) -> Bus Creator/8
  RotoTestEthRX/23(WatchdogCnt) -> Bus Creator/23
  RotoTestEthRX/18(RefRR_Nm) -> Bus Creator/18
  Mux1/1 -> SpdAct/1
  RotoTestEthRX/19(UnitsStatusLF) -> Bus Creator/19
  RotoTestEthRX/4(ActSpLF_rpm) -> Bus Creator/4
  Bus Creator/1 -> AxlTrq/1, Bus Selector1/1
  Bus Selector1/4 -> Mux1/4  "<ActSpRR_rpm>"
  RotoTestEthRX/24(FaultActive) -> Bus Creator/24
  RotoTestEthRX/22(UnitsStatusRR) -> Bus Creator/22
  Bus Selector1/3 -> Mux1/3  "<ActSpLR_rpm>"
  RotoTestEthRX/25(WarningsActive) -> Bus Creator/25
  Bus Selector1/1 -> Mux1/1  "<ActSpLF_rpm>"
  Bus Selector1/2 -> Mux1/2  "<ActSpRF_rpm>"
  RotoTestEthRX/5(ActTempLF_C) -> Bus Creator/5
  RotoTestEthRX/30(SystemActive) -> Bus Creator/30
  RotoTestEthRX/20(UnitsStatusRF) -> Bus Creator/20
  RotoTestEthRX/15(RefLF_Nm) -> Bus Creator/15
  RotoTestEthRX/16(RefRF_rpm) -> Bus Creator/16
  RotoTestEthRX/17(RefLR_Nm) -> Bus Creator/17
  RotoTestEthRX/2(ProtocolVer) -> Bus Creator/2
  RotoTestEthRX/7(ActSpRF_rpm) -> Bus Creator/7
  RotoTestEthRX/21(UnitsStatusLR) -> Bus Creator/21
  RotoTestEthRX/11(ActTempLR_C) -> Bus Creator/11
  RotoTestEthRX/1(ID) -> Bus Creator/1
  RotoTestEthRX/28(SpTqRF) -> Bus Creator/28
  RotoTestEthRX/29(SpTqLF) -> Bus Creator/29
  RotoTestEthRX/27(SpTqLR) -> Bus Creator/27
  RotoTestEthRX/26(SpTqRR) -> Bus Creator/26
  RotoTestEthRX/14(ActTempRR_Nm) -> Bus Creator/14
  RotoTestEthRX/3(ActTqLF_Nm) -> Bus Creator/3
  RotoTestEthRX/6(ActTqRF_Nm_) -> Bus Creator/6
  RotoTestEthRX/9(ActTqLR_Nm) -> Bus Creator/9
  RotoTestEthRX/13(ActSpRR_rpm) -> Bus Creator/13
  RotoTestEthRX/10(ActSpLR_rpm) -> Bus Creator/10
  RotoTestEthRX/12(ActTqRR_Nm) -> Bus Creator/12
  Input/1 -> RotoTestEthRX/1(Input)

== system CAVE_MachE/Vehicle Under Test/Vehicle/Rototest and ORNL Interface/Get Wheel Spd Cmd Based on Wheel Dynamics ==
  BrakingTorques : Inport
  Trq_T2W : Inport  Port=2
  AxlTrq : Inport  Port=3
  MaxRegen : Inport  Port=4
  FxIn : Inport  Port=5
  Saturation : Saturate  UpperLimit=100  LowerLimit=0
  Saturation1 : Saturate  UpperLimit=300  LowerLimit=-300
  Scope : Scope
  WheelSpdCmd : Subsystem
  Whl Dynamics & Format CM Powertrain Signal : Subsystem
  WhlSpdCmd : Outport
  wires:
  Whl Dynamics & Format CM Powertrain Signal/1(PowerTrainOutIdeal) -> WheelSpdCmd/1(In1)
  BrakingTorques/1 -> Whl Dynamics & Format CM Powertrain Signal/1(BrakingTorques)
  Trq_T2W/1 -> Whl Dynamics & Format CM Powertrain Signal/2(Trq_T2W)
  MaxRegen/1 -> Whl Dynamics & Format CM Powertrain Signal/4(MaxRegen)
  AxlTrq/1 -> Whl Dynamics & Format CM Powertrain Signal/3(AxlTrq)
  FxIn/1 -> Whl Dynamics & Format CM Powertrain Signal/5(FxIn)
  [SimOmega] -> Scope/1, Saturation/1
  Saturation/1 -> WhlSpdCmd/1

== system CAVE_MachE/Vehicle Under Test/Vehicle/Rototest and ORNL Interface/RotoTrqPreprocess ==
  AxleTrqRaw : Inport
  Bus Selector1 : BusSelector  OutputSignals=ActTqLF_Nm_,ActTqRF_Nm_,ActTqLR_Nm_,ActTqRR_Nm_
  Compare To Constant : simulink/Logic and Bit Operations/Compare To Constant  relop=>=  const=-15  OutDataTypeStr=boolean
  Compare To Constant1 : simulink/Logic and Bit Operations/Compare To Constant  relop=<=  const=0  OutDataTypeStr=boolean
  Data Type Conversion{1..4} (4 alike) : DataTypeConversion  OutDataTypeStr=double  SaturateOnIntegerOverflow=off  RndMeth=Floor
  FirstOrderFilterTau{,1..3} (4 alike) : VSIGenLib/FirstOrderFilterTau  SystemSampleTime=-1  VariantActivationTime=update diagram  AllowFlexibleInterface=on  Latency=0  AutoFrameSizeCalculation=off
  Ground : Ground
  Logical Operator : Logic  AllPortsSameDT=off  OutDataTypeStr=boolean
  ManualTrq_Nm : Constant  Value=0
  Mux : Mux
  Mux1 : Mux
  SatTrq : Saturate  UpperLimit=1000  LowerLimit=-1000
  Tau : Constant  Value=0.01
  TorqueIn : Switch  Criteria=u2 > Threshold  SaturateOnIntegerOverflow=off  InputSameDT=off
  "TorqueIn " : Switch  Criteria=u2 > Threshold  SaturateOnIntegerOverflow=off  InputSameDT=off
  AxleTrqRoto : Outport
  AxleTrqVeh : Outport  Port=2
  wires:
  Mux/1 -> AxleTrqRoto/1, TorqueIn/1
  ManualTrq_Nm/1 -> Mux1/4, Mux1/3, Mux1/2, Mux1/1
  Tau/1 -> FirstOrderFilterTau/2, FirstOrderFilterTau1/2, FirstOrderFilterTau2/2, FirstOrderFilterTau3/2
  Ground/1 -> "TorqueIn "/1
  Logical Operator/1 -> "TorqueIn "/2
  Data Type Conversion4/1 -> Mux/4  "RR"
  Data Type Conversion3/1 -> Mux/3  "LR"
  Mux1/1 -> TorqueIn/3
  [Switch] -> TorqueIn/2
  Bus Selector1/4 -> FirstOrderFilterTau3/1  "<ActTqRR_Nm_>"
  Compare To Constant/1 -> Logical Operator/1
  Bus Selector1/3 -> FirstOrderFilterTau2/1  "<ActTqLR_Nm_>"
  Bus Selector1/2 -> FirstOrderFilterTau1/1  "<ActTqRF_Nm_>"
  TorqueIn/1 -> SatTrq/1
  "TorqueIn "/1 -> AxleTrqVeh/1  "Trq"
  FirstOrderFilterTau1/1 -> Data Type Conversion2/1
  Data Type Conversion2/1 -> Mux/2  "RF"
  AxleTrqRaw/1 -> Bus Selector1/1
  FirstOrderFilterTau/1 -> Data Type Conversion1/1
  FirstOrderFilterTau3/1 -> Data Type Conversion4/1
  Bus Selector1/1 -> FirstOrderFilterTau/1  "<ActTqLF_Nm_>"
  Compare To Constant1/1 -> Logical Operator/2
  SatTrq/1 -> "TorqueIn "/3, Compare To Constant1/1, Compare To Constant/1
  FirstOrderFilterTau2/1 -> Data Type Conversion3/1
  Data Type Conversion1/1 -> Mux/1  "LF"

== system CAVE_MachE/Vehicle Under Test/Vehicle/Rototest and ORNL Interface/Subsystem2 ==
  AxlTorq : Inport
  BusCreator1 : BusCreator  Inputs=16
  BusCreator2 : BusCreator  Inputs=16
  Constant : Constant  Value=0
  Constant1 : Constant  Value=0
  Demux : Demux  Outputs=16
      settings: DisplayOption=none
  Terminator : Terminator
  Zero1 : Constant  Value=0
  Zero2 : Constant  Value=0
  Zero5 : Constant  Value=0
  BrakeUpd : Outport
  wires:
  Demux/9 -> BusCreator1/9  "Brake IF Trq_Reg_trg FL"
  Demux/6 -> BusCreator1/6  "Brake IF Trq_PB FR"
  Constant1/1 -> BusCreator2/1, BusCreator2/2  "Brake IF Trq_WB FL"
  Demux/14 -> BusCreator1/14  "Brake IF Trq_DriveSrc_trg d1"
  Zero2/1 -> BusCreator2/16, BusCreator2/15, BusCreator2/14, BusCreator2/13  "Brake IF Trq_DriveSrc_trg d3"
  Demux/11 -> BusCreator1/11  "Brake IF Trq_Reg_trg RL"
  Demux/15 -> BusCreator1/15  "Brake IF Trq_DriveSrc_trg d2"
  Demux/2 -> BusCreator1/2  "Brake IF Trq_WB FR"
  Demux/16 -> BusCreator1/16  "Brake IF Trq_DriveSrc_trg d3"
  Zero1/1 -> BusCreator2/12, BusCreator2/11, BusCreator2/10, BusCreator2/9  "Brake IF Trq_Reg_trg RR"
  Demux/4 -> BusCreator1/4  "Brake IF Trq_WB RR"
  Demux/3 -> BusCreator1/3  "Brake IF Trq_WB RL"
  Constant/1 -> BusCreator2/4, BusCreator2/3  "Brake IF Trq_WB RL"
  BusCreator1/1 -> BrakeUpd/1
  Demux/1 -> BusCreator1/1  "Brake IF Trq_WB FL"
  Demux/8 -> BusCreator1/8  "Brake IF Trq_PB RR"
  Demux/10 -> BusCreator1/10  "Brake IF Trq_Reg_trg FR"
  BusCreator2/1 -> Demux/1
  Demux/13 -> BusCreator1/13  "Brake IF Trq_DriveSrc_trg d0"
  Demux/5 -> BusCreator1/5  "Brake IF Trq_PB FL"
  Demux/7 -> BusCreator1/7  "Brake IF Trq_PB RL"
  Zero5/1 -> BusCreator2/8, BusCreator2/7, BusCreator2/6, BusCreator2/5  "Brake IF Trq_PB RR"
  Demux/12 -> BusCreator1/12  "Brake IF Trq_Reg_trg RR"
  AxlTorq/1 -> Terminator/1

== system CAVE_MachE/Vehicle Under Test/Vehicle/Rototest and ORNL Interface/To Rototest with Band-Aid ==
  note: Torque Model: Low speed
      | Speed Model: Normal speed
  note: OutMode = 0 is Torque
      | OutMode = 1 is Speed
  note: Switch = 0 Overides
      | Switch = 1 Model
  SpeedCmd_rps : Inport
  AxleTrq_roto_Nm : Inport  Port=2
  BRAKE_PRESSED : Inport  Port=3
  Vehicle_Speed_kph : Inport  Port=4
  Band-Aid : Subsystem
  Demux : Demux
  Demux1 : Demux
  Demux2 : Demux
  Logging : Subsystem  Commented=on
  MasterSw : Constant  Value=0
  Mode Override : Subsystem
  ModeOut : Switch  Criteria=u2 > Threshold  SaturateOnIntegerOverflow=off  InputSameDT=off
  ModeSwitch : MultiPortSwitch  DataPortOrder=Zero-based contiguous  Inputs=2  zeroidx=on  SaturateOnIntegerOverflow=off  InputSameDT=off
  Mux2 : Mux
  Mux4 : Mux
  Mux5 : Mux
  RateLimSpd : RateLimiter  RisingSlewLimit=500  FallingSlewLimit=-500  SampleTimeMode=inherited
  RotoTestEthTx : Subsystem  AncestorBlock=VSIGenLib/RotoTestEthTx
      mask Display:
      | color('white')
      | disp('RotTestEthTx')
      | port_label('input', 1, 'RefLF_NmORrpm')
      | port_label('input', 2, 'RefRF_NmORrpm')
      | port_label('input', 3, 'RefLR_NmORrpm')
      | port_label('input', 4, 'RefRR_NmORrpm')
      | port_label('input', 5, 'SqTrRR')
      | port_label('input', 6, 'SqTrLR')
      | port_label('input', 7, 'SqTrRF')
      | port_label('input', 8, 'SqTrLF')
      | port_label('input', 9, 'SystemActive')
      | port_label('output', 1, 'Status (bool)')
      | port_label('output', 2, 'Sent Bytes (int)')
  SatSpd : Saturate  UpperLimit=500  LowerLimit=0
  Scope : Scope
  SpeedOut : Switch  Criteria=u2 > Threshold  SaturateOnIntegerOverflow=off  InputSameDT=off
  SystemActive : Constant  Value=0  OutDataTypeStr=uint8
  Transfer Fcn{,1..3} (4 alike) : TransferFcn  Denominator=[0.02 1]
  TrqSpd Override : Subsystem
  ZeroTorque : Constant  Value=0  OutDataTypeStr=uint8
  rads2rpm : Gain  Gain=9.5492965964254
  Out1 : Outport
  tag scope: Switch=global
  wires:
  Mux4/1 -> ModeSwitch/2
  Demux/3 -> Mux2/3  "LRIn"
  Demux1/4 -> Transfer Fcn3/1
  Demux/2 -> Mux2/2  "RFIn"
  MasterSw/1 -> [Switch]
  TrqSpd Override/1(Ovr) -> SpeedOut/3
  ZeroTorque/1 -> Mux4/2, Mux4/3, Mux4/4, Mux4/1
  Demux/1 -> Mux2/1  "LFIn"
  SpeedOut/1 -> RateLimSpd/1
  RateLimSpd/1 -> SatSpd/1
  rads2rpm/1 -> Demux/1
  ModeSwitch/1 -> Scope/1, Demux1/1
  Demux/4 -> Mux2/4  "RRIn"
  Band-Aid/1(OutMode) -> Mux5/4, Mux5/3, Mux5/2, Mux5/1, ModeSwitch/1
  ModeOut/1 -> Demux2/1
  [Switch] -> SpeedOut/2
  SatSpd/1 -> ModeSwitch/3  "Spd"
  [Switch] -> ModeOut/2
  Mux5/1 -> ModeOut/1
  Demux2/1 -> RotoTestEthTx/5(SpTqRR)
  Demux1/3 -> Transfer Fcn2/1
  Demux2/3 -> RotoTestEthTx/7(SpTqRF)
  Demux2/2 -> RotoTestEthTx/6(SpTqLR)
  SystemActive/1 -> RotoTestEthTx/9(SystemActive)
  RotoTestEthTx/1(Output) -> Out1/1  "ByteSend"
  Demux1/1 -> Transfer Fcn/1
  Demux1/2 -> Transfer Fcn1/1
  Demux2/4 -> RotoTestEthTx/8(SpTqLF)
  SpeedCmd_rps/1 -> rads2rpm/1
  Mode Override/1(Ovr) -> ModeOut/3
  AxleTrq_roto_Nm/1 -> Band-Aid/2(InTrq_Nm)
  Mux2/1 -> Band-Aid/1(InSpd_rpm)
  Band-Aid/2(OutSpd_rpm) -> SpeedOut/1
  BRAKE_PRESSED/1 -> Band-Aid/3(BRAKE_PRESSED)
  Vehicle_Speed_kph/1 -> Band-Aid/4(VehSpd_kph)
  Transfer Fcn/1 -> RotoTestEthTx/1(RefLF_NmORrpm)
  Transfer Fcn1/1 -> RotoTestEthTx/2(RefRF_NmORrpm)
  Transfer Fcn2/1 -> RotoTestEthTx/3(RefLR_NmORrpm)
  Transfer Fcn3/1 -> RotoTestEthTx/4(RefRR_NmORrpm)

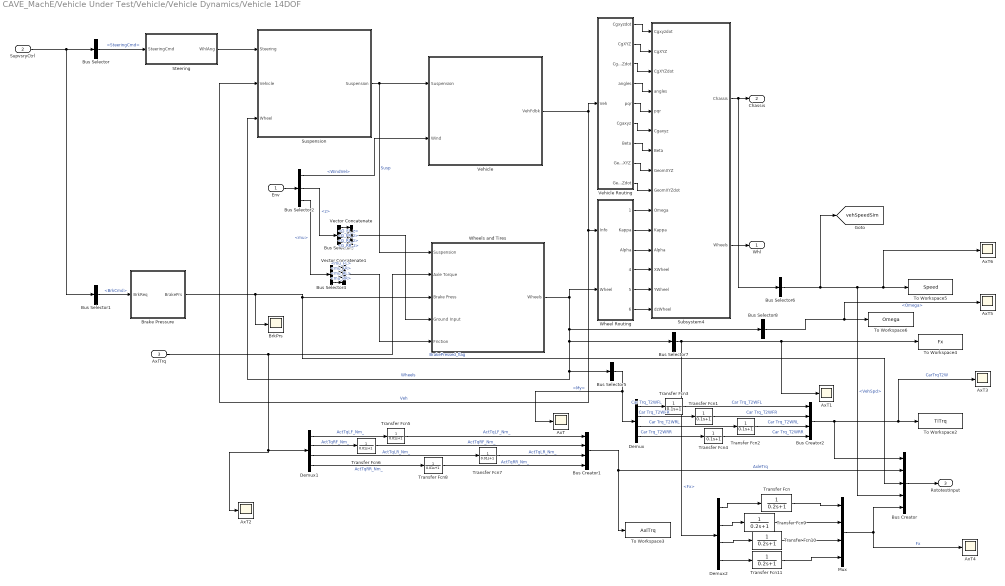
== system CAVE_MachE/Vehicle Under Test/Vehicle/Vehicle Dynamics/Vehicle 14DOF ==
  Env : Inport
  SupvsryCtrl : Inport  Port=2
  AxlTrq : Inport  Port=3
  AxT{,1..6} (7 alike) : Scope
  Brake Pressure : Subsystem
  BrkPrs : Scope
  Bus Creator : BusCreator  Inputs=5
  Bus Creator1 : BusCreator  Inputs=ActTqLF_Nm_,ActTqRF_Nm_,ActTqLR_Nm_,ActTqRR_Nm_
  Bus Creator2 : BusCreator  Inputs=Car Trq_T2WFL,Car Trq_T2WFR,Car Trq_T2WRL,Car Trq_T2WRR
  Bus Selector : BusSelector  OutputSignals=SteeringCmd
  Bus Selector1 : BusSelector  OutputSignals=BrkCmd
  Bus Selector2 : BusSelector  OutputSignals=WindVel,GndBus.z,GndBus.mu
  Bus Selector3 : BusSelector  OutputSignals=G_FL_z,G_FR_z,G_RL_z,G_RR_z
  Bus Selector4 : BusSelector  OutputSignals=mu_FL,mu_FR,mu_RL,mu_RR
  Bus Selector5 : BusSelector  OutputSignals=TireFrame.My
  Bus Selector6 : BusSelector  OutputSignals=VehSpd
  Bus Selector7 : BusSelector  OutputSignals=TireFrame.Fx
  Bus Selector8 : BusSelector  OutputSignals=TireFrame.Omega
  Demux : Demux
  Demux1 : Demux
  Demux2 : Demux
  Mux : Mux
  Steering : Subsystem
  Subsystem4 : Subsystem
  Suspension : Subsystem  Variant=on  VariantControlMode=label  LabelModeActiveChoice=3
      mask Display:
      | switch str2num(get_param(gcb,'ActiveVariant'))
      |     case 1
      |         image('suspdw.png');
      |     case 2
      |         image([imread('suspindmap.png');imread('suspsamap.png')]);
      |     case 3
      |          image([imread('suspmacp.png');imread('suspsacoil.png')]);
      |     case 4
      |          image('suspmacp.png');
      |     case 5
      |          image('suspindmap.png');
      | end
  To Workspace2 : ToWorkspace  VariableName=TiTrq  SampleTime=-1
      settings: Save2DSignal=2-D array (concatenate along first dimension)
  To Workspace3 : ToWorkspace  VariableName=AxlTrq  SampleTime=-1
      settings: Save2DSignal=2-D array (concatenate along first dimension)
  To Workspace4 : ToWorkspace  VariableName=Fx  SampleTime=-1
      settings: Save2DSignal=2-D array (concatenate along first dimension)
  To Workspace5 : ToWorkspace  VariableName=Speed  SampleTime=-1
      settings: Save2DSignal=2-D array (concatenate along first dimension)
  To Workspace6 : ToWorkspace  VariableName=Omega  SampleTime=-1
      settings: Save2DSignal=2-D array (concatenate along first dimension)
  Transfer Fcn{,9..11} (4 alike) : TransferFcn  Denominator=[0.2 1]
  Transfer Fcn{1..4} (4 alike) : TransferFcn  Denominator=[0.1 1]
  Transfer Fcn{5..8} (4 alike) : TransferFcn  Denominator=[0.01 1]
  Vector Concatenate : Concatenate  NumInputs=4
  Vector Concatenate1 : Concatenate  NumInputs=4
  Vehicle : Subsystem
      mask Display: image('6dofcar.png');
  Vehicle Routing : Subsystem
  Wheel Routing : Subsystem
  Wheels and Tires : Subsystem
      mask Display: image('wheel3dof.png')
  Whl : Outport
  Chassis : Outport  Port=2
  RototestInput : Outport  Port=3
  tag scope: vehSpeedSim=global
  wires:
  Vehicle Routing/9(GeomXYZdot) -> Subsystem4/9(GeomXYZdot)
  Vehicle Routing/8(GeomXYZ) -> Subsystem4/8(GeomXYZ)
  Vehicle Routing/1(Cgxyzdot) -> Subsystem4/1(Cgxyzdot)
  Vehicle Routing/5(pqr) -> Subsystem4/5(pqr)
  Vehicle Routing/4(angles) -> Subsystem4/4(angles)
  Vehicle Routing/3(CgXYZdot) -> Subsystem4/3(CgXYZdot)
  Vehicle Routing/7(Beta) -> Subsystem4/7(Beta)
  Wheels and Tires/1(Wheels) -> Wheel Routing/2(Wheel), Bus Selector7/1, Bus Selector5/1, Suspension/3(Wheel), Bus Selector8/1  "Wheels"
  Vehicle Routing/2(CgXYZ) -> Subsystem4/2(CgXYZ)
  Vehicle/1(VehFdbk) -> Suspension/2(Vehicle), Wheel Routing/1(Info), Vehicle Routing/1(Veh)  "Veh"
  Suspension/1(Suspension) -> Vehicle/1(Suspension), Wheels and Tires/1(Suspension)  "Susp"
  Bus Selector2/1 -> Vehicle/2(Wind)  "<WindVel>"
  Steering/1(WhlAng) -> Suspension/1(Steering)
  Bus Selector/1 -> Steering/1(SteeringCmd)  "<SteeringCmd>"
  SupvsryCtrl/1 -> Bus Selector/1, Bus Selector1/1
  Bus Selector1/1 -> Brake Pressure/1(BrkReq)  "<BrkCmd>"
  Env/1 -> Bus Selector2/1
  Vehicle Routing/6(Cgaxyz) -> Subsystem4/6(Cgaxyz)
  Wheel Routing/1(Omega) -> Subsystem4/10(Omega)
  Wheel Routing/3(Alpha) -> Subsystem4/12(Alpha)
  Wheel Routing/4(XWheel) -> Subsystem4/13(XWheel)
  Wheel Routing/2(Kappa) -> Subsystem4/11(Kappa)
  Wheel Routing/5(YWheel) -> Subsystem4/14(YWheel)
  Wheel Routing/6(ZWheel) -> Subsystem4/15(dzWheel)
  Subsystem4/2(Wheels) -> Whl/1
  AxlTrq/1 -> Demux1/1, AxT2/1, Wheels and Tires/2(Axle Torque)
  Bus Selector2/2 -> Bus Selector3/1  "<z>"
  Bus Selector3/1 -> Vector Concatenate/1  "<G_FL_z>"
  Bus Selector3/2 -> Vector Concatenate/2  "<G_FR_z>"
  Bus Selector3/3 -> Vector Concatenate/3  "<G_RL_z>"
  Bus Selector3/4 -> Vector Concatenate/4  "<G_RR_z>"
  Vector Concatenate/1 -> Wheels and Tires/4(Ground Input)
  Bus Selector4/4 -> Vector Concatenate1/4  "<mu_RR>"
  Bus Selector2/3 -> Bus Selector4/1  "<mu>"
  Bus Selector4/3 -> Vector Concatenate1/3  "<mu_RL>"
  Bus Selector4/2 -> Vector Concatenate1/2  "<mu_FR>"
  Bus Selector4/1 -> Vector Concatenate1/1  "<mu_FL>"
  Vector Concatenate1/1 -> Wheels and Tires/5(Friction)
  Bus Selector6/1 -> [vehSpeedSim], Bus Creator/4, AxT6/1, To Workspace5/1  "<VehSpd>"
  Brake Pressure/1(BrakePrs) -> BrkPrs/1, Bus Creator/3, Wheels and Tires/3(Brake Press)  "BrakePressed_flag"
  Bus Creator1/1 -> To Workspace3/1, Bus Creator/2  "AxleTrq"
  Bus Creator2/1 -> Bus Creator/1, AxT3/1, To Workspace2/1  "CarTrqT2W"
  Bus Selector5/1 -> Demux/1, AxT/1  "<My>"
  Subsystem4/1(Chassis) -> Bus Selector6/1, Chassis/1
  Bus Selector7/1 -> Demux2/1, AxT1/1, To Workspace4/1  "<Fx>"
  Bus Selector8/1 -> AxT5/1, To Workspace6/1  "<Omega>"
  Bus Creator/1 -> RototestInput/1
  Transfer Fcn5/1 -> Bus Creator1/1  "ActTqLF_Nm_"
  Demux1/3 -> Transfer Fcn7/1  "ActTqLR_Nm_"
  Transfer Fcn8/1 -> Bus Creator1/4  "ActTqRR_Nm_"
  Demux1/2 -> Transfer Fcn6/1  "ActTqRF_Nm_"
  Transfer Fcn6/1 -> Bus Creator1/2  "ActTqRF_Nm_"
  Demux1/1 -> Transfer Fcn5/1  "ActTqLF_Nm_"
  Transfer Fcn7/1 -> Bus Creator1/3  "ActTqLR_Nm_"
  Demux1/4 -> Transfer Fcn8/1  "ActTqRR_Nm_"
  Demux2/3 -> Transfer Fcn10/1
  Transfer Fcn10/1 -> Mux/3
  Demux2/2 -> Transfer Fcn9/1
  Transfer Fcn9/1 -> Mux/2
  Demux2/4 -> Transfer Fcn11/1
  Transfer Fcn/1 -> Mux/1
  Demux2/1 -> Transfer Fcn/1
  Transfer Fcn11/1 -> Mux/4
  Mux/1 -> AxT4/1, Bus Creator/5  "Fx"
  Transfer Fcn3/1 -> Bus Creator2/1  "Car Trq_T2WFL"
  Demux/3 -> Transfer Fcn2/1  "Car Trq_T2WRL"
  Transfer Fcn1/1 -> Bus Creator2/2  "Car Trq_T2WFR"
  Demux/2 -> Transfer Fcn1/1  "Car Trq_T2WFR"
  Demux/1 -> Transfer Fcn3/1  "Car Trq_T2WFL"
  Demux/4 -> Transfer Fcn4/1  "Car Trq_T2WRR"
  Transfer Fcn4/1 -> Bus Creator2/4  "Car Trq_T2WRR"
  Transfer Fcn2/1 -> Bus Creator2/3  "Car Trq_T2WRL"
